simulink model "pendubotG_PID_FUNZY"  (R2017b)
settings: Solver=FixedStepAuto  StartTime=0.0  StopTime=10  FixedStep=0.01  RelTol=1e-3
values from neighbouring files (symbols this model uses):
  Kd1 = par(bestchrom,3)-500    [pidGA.m]    (also in thongso_pid_chuan.m = -214.2; thongso_pid_chuan_phuc_chay.m = -315.3)
  Kp1 = par(bestchrom,1)-500    [pidGA.m]    (also in thongso_pid_chuan.m = -416.5; thongso_pid_chuan_phuc_chay.m = -885.5)
  q1_d_init = 0.0001    [goc_init.m]
  q1_init = pi/2+0.001    (= 1.57179632679)    [goc_init.m]
  q2_d_init = 0.02    [goc_init.m]
  q2_init = 0.007    [goc_init.m]
libraries: fuzblock x4
settings Model: Creator=vohuu  LastModifiedBy=DELL
settings DebuggingCC: UnconnectedInputMsg=none  UnconnectedOutputMsg=none  UnconnectedLineMsg=none  SFMachineParentedDataDiag=error
settings SFSimCC: SimUseLocalCustomCode=on
settings RTWCC: RTWUseLocalCustomCode=on
settings CodeAppCC: StateflowObjectComments=on

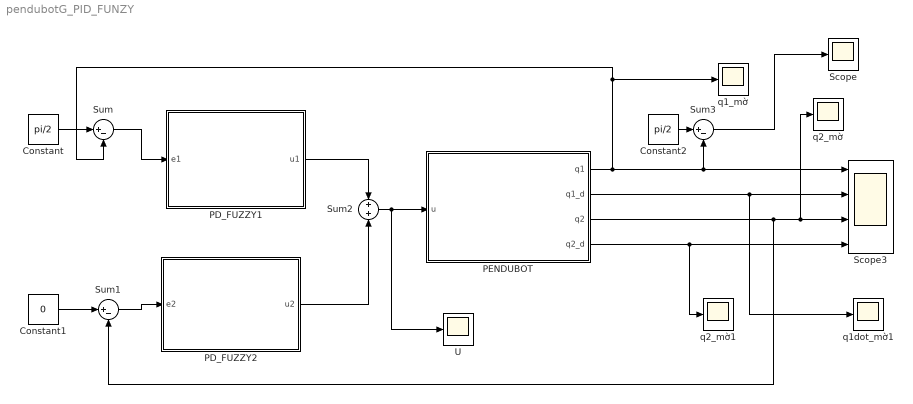
== system pendubotG_PID_FUNZY ==
  Constant : Constant  Value=pi/2
  Constant1 : Constant  Value=0
  Constant2 : Constant  Value=pi/2
  PD_FUZZY1 : Subsystem
  PD_FUZZY2 : Subsystem
  PENDUBOT : Subsystem
  Scope : Scope
  Scope3 : Scope  NumInputPorts=4
  Sum : Sum  Inputs=|+-
  Sum1 : Sum  Inputs=|+-
  Sum2 : Sum
  Sum3 : Sum  Inputs=|+-
  "U " : Scope
  q1_mờ : Scope
  q1dot_mờ1 : Scope
  q2_mờ : Scope
  q2_mờ1 : Scope
  wires:
  Sum1/1 -> PD_FUZZY2/1(e2)
  PD_FUZZY2/1(u2) -> Sum2/2
  Constant1/1 -> Sum1/1
  Sum/1 -> PD_FUZZY1/1(e1)
  PENDUBOT/4(q2_d) -> q2_mờ1/1, Scope3/4
  Sum2/1 -> "U "/1, PENDUBOT/1(u)
  PENDUBOT/2(q1_d) -> q1dot_mờ1/1, Scope3/2
  Constant/1 -> Sum/1
  PENDUBOT/3(q2) -> q2_mờ/1, Scope3/3, Sum1/2
  PENDUBOT/1(q1) -> Scope3/1, Sum3/2, Sum/2, q1_mờ/1
  Constant2/1 -> Sum3/1
  PD_FUZZY1/1(u1) -> Sum2/1
  Sum3/1 -> Scope/1

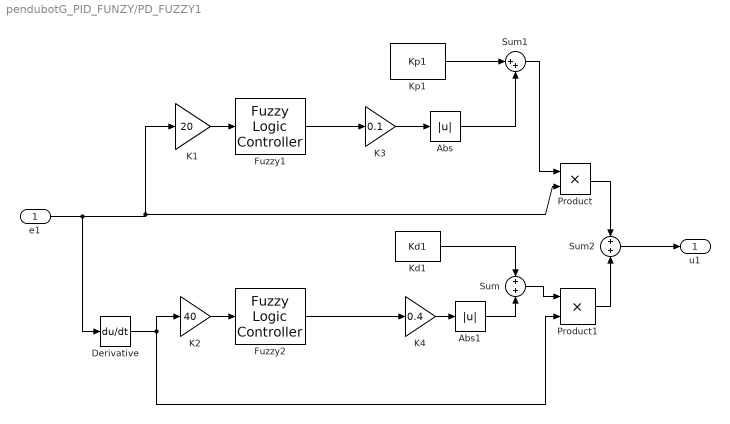
== system pendubotG_PID_FUNZY/PD_FUZZY1 ==
  e1 : Inport
  Abs : Abs
  Abs1 : Abs
  Derivative : Derivative
  "Fuzzy1 " : fuzblock/Fuzzy Logic  Controller  FIS='RULE111.fis'  OutputSampleNumber=101  DataType=double  FuzzifiedInputs=off  RuleFiringStrengths=off  RuleOutputs=off  AggregatedOutputs=off  SimulateUsing=Interpreted execution
  Fuzzy2 : fuzblock/Fuzzy Logic  Controller  FIS='RULE222.fis'  OutputSampleNumber=101  DataType=double  FuzzifiedInputs=off  RuleFiringStrengths=off  RuleOutputs=off  AggregatedOutputs=off  SimulateUsing=Interpreted execution
  K1 : Gain  Gain=20
  K2 : Gain  Gain=40
  K3 : Gain  Gain=0.1
  K4 : Gain  Gain=0.4
  Kd1 : Constant  Value=Kd1
  Kp1 : Constant  Value=Kp1
  Product : Product
  Product1 : Product
  Sum : Sum
  Sum1 : Sum  Inputs=|++
  Sum2 : Sum
  u1 : Outport
  wires:
  K1/1 -> "Fuzzy1 "/1
  "Fuzzy1 "/1 -> K3/1
  K3/1 -> Abs/1
  Kp1/1 -> Sum1/1
  Sum1/1 -> Product/1
  e1/1 -> K1/1, Product/2, Derivative/1
  Abs/1 -> Sum1/2
  K2/1 -> Fuzzy2/1
  Derivative/1 -> Product1/2, K2/1
  Fuzzy2/1 -> K4/1
  Kd1/1 -> Sum/1
  K4/1 -> Abs1/1
  Abs1/1 -> Sum/2
  Sum/1 -> Product1/1
  Product1/1 -> Sum2/2
  Product/1 -> Sum2/1
  Sum2/1 -> u1/1

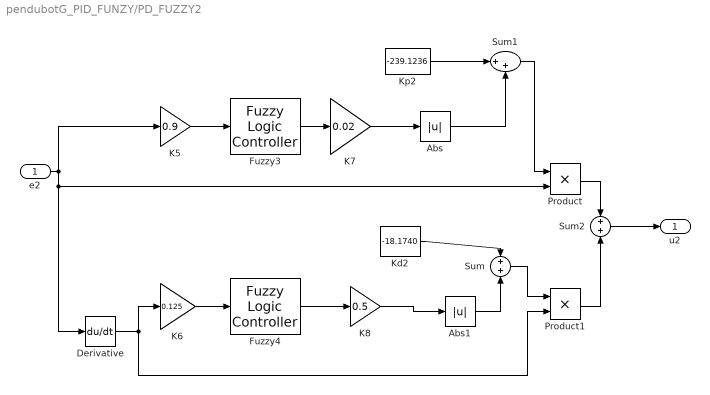
== system pendubotG_PID_FUNZY/PD_FUZZY2 ==
  e2 : Inport
  Abs : Abs
  Abs1 : Abs
  Derivative : Derivative
  Fuzzy3 : fuzblock/Fuzzy Logic  Controller  FIS='RULE333.fis'  OutputSampleNumber=101  DataType=double  FuzzifiedInputs=off  RuleFiringStrengths=off  RuleOutputs=off  AggregatedOutputs=off  SimulateUsing=Interpreted execution
  Fuzzy4 : fuzblock/Fuzzy Logic  Controller  FIS='RULE444.fis'  OutputSampleNumber=101  DataType=double  FuzzifiedInputs=off  RuleFiringStrengths=off  RuleOutputs=off  AggregatedOutputs=off  SimulateUsing=Interpreted execution
  K5 : Gain  Gain=0.9
  K6 : Gain  Gain=0.125
  K7 : Gain  Gain=0.02
  K8 : Gain  Gain=0.5
  Kd2 : Constant  Value=-18.1740
  Kp2 : Constant  Value=-239.1236
  Product : Product
  Product1 : Product
  Sum : Sum
  Sum1 : Sum  Inputs=|++
  Sum2 : Sum
  u2 : Outport
  wires:
  Sum2/1 -> u2/1
  Product/1 -> Sum2/1
  Product1/1 -> Sum2/2
  Sum/1 -> Product1/1
  Abs1/1 -> Sum/2
  K8/1 -> Abs1/1
  Kd2/1 -> Sum/1
  Fuzzy4/1 -> K8/1
  Derivative/1 -> Product1/2, K6/1
  K6/1 -> Fuzzy4/1
  Abs/1 -> Sum1/2
  e2/1 -> Derivative/1, Product/2, K5/1
  Sum1/1 -> Product/1
  Kp2/1 -> Sum1/1
  K7/1 -> Abs/1
  Fuzzy3/1 -> K7/1
  K5/1 -> Fuzzy3/1

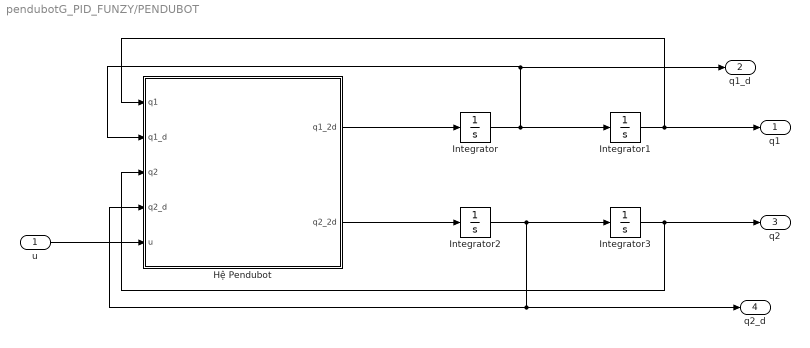
== system pendubotG_PID_FUNZY/PENDUBOT ==
  u : Inport
  Hệ Pendubot : MATLAB Function  TreatAsAtomicUnit=on
  Integrator : Integrator  InitialCondition=q1_d_init
  Integrator1 : Integrator  InitialCondition=q1_init
  Integrator2 : Integrator  InitialCondition=q2_d_init
  Integrator3 : Integrator  InitialCondition=q2_init
  q1 : Outport
  q1_d : Outport  Port=2
  q2 : Outport  Port=3
  q2_d : Outport  Port=4
  wires:
  Integrator2/1 -> q2_d/1, Hệ Pendubot/4(q2_d), Integrator3/1
  Integrator3/1 -> Hệ Pendubot/3(q2), q2/1
  Integrator/1 -> Hệ Pendubot/2(q1_d), q1_d/1, Integrator1/1
  u/1 -> Hệ Pendubot/5(u)
  Hệ Pendubot/2(q2_2d) -> Integrator2/1
  Integrator1/1 -> Hệ Pendubot/1(q1), q1/1
  Hệ Pendubot/1(q1_2d) -> Integrator/1

== matlab function pendubotG_PID_FUNZY/PENDUBOT/Hệ Pendubot ==
  data: q1 input; q1_2d output; q1_d input; q2 input; q2_d input; u input; q2_2d output
function [q1_2d,q2_2d] = fcn(q1,q1_d,q2,q2_d,u)
m1=1.068;
m2=0.07;
l1=0.146;
l2=0.253;
lc1=0.055;
lc2=0.149;
I1=0.0189;
I2=0.000409;
Kb=0.0864;
Kt=0.0864;
Rm=3.7;
Cm=0.000415;
Jm=0.000427;
g=9.80665;
K1=Kt/Rm;
K2=((Kt*Kb)/Rm)+Cm;
K3=Jm;
beta1=m1*lc1^2+m2*l1^2+I1;
beta2=m2*lc2^2+I2;
beta3=m2*l1*lc2;
beta4=m1*lc1+m2*l1;
beta5=m2*lc2;
q1_2d=1/(beta1*beta2-beta3^2*(cos(q2))^2+K3*beta2)*(beta2*beta3*sin(q2)*(q1_d+q2_d)^2+beta3^2*cos(q2)*sin(q2)*q1_d^2-beta2*beta4*g*cos(q1)+beta3*beta5*g*cos(q2)*cos(q1+q2)+beta2*K1*u-K2*beta2*q1_d);
%q2_2d=-(2*beta3^2*q1_d^2*sin(2*q2) + beta3^2*q2_d^2*sin(2*q2) - 2*K2*beta2*q1_d + 2*K1*beta2*u + 2*K3*beta5*g*cos(q1 + q2) + 2*beta1*beta5*g*cos(q1 + q2) - beta3*beta4*g*cos(q1 + q2) + 2*beta3^2*q1_d*q2_d*sin(2*q2) - 2*K2*beta3*q1_d*cos(q2) + 2*K1*beta3*u*cos(q2) - 2*beta2*beta4*g*cos(q1) + beta3*beta5*g*cos(q1) - beta3*beta4*g*cos(q1 - q2) + beta3*beta5*g*cos(q1 + 2*q2) + 2*K3*beta3*q1_d^2*sin(q2) + 2*beta1*beta3*q1_d^2*sin(q2) + 2*beta2*beta3*q1_d^2*sin(q2) + 2*beta2*beta3*q2_d^2*sin(q2) + 4*beta2*beta3*q1_d*q2_d*sin(q2))/(2*K3*beta2 + 2*beta1*beta2 - beta3^2*cos(2*q2) - beta3^2);
q2_2d=-(beta5*g*cos(q1 + q2)*(K3 + beta1 + beta3*cos(q2)) - beta4*g*cos(q1)*(beta2 + beta3*cos(q2)) - K2*q1_d*(beta2 + beta3*cos(q2)) + beta3*sin(q2)*(q1_d + q2_d)^2*(beta2 + beta3*cos(q2)) + K3*beta3*q1_d^2*sin(q2) + beta3*q1_d^2*sin(q2)*(beta1 + beta3*cos(q2)))/(- beta3^2*cos(q2)^2 + K3*beta2 + beta1*beta2) - (K1*u*(beta2 + beta3*cos(q2)))/(- beta3^2*cos(q2)^2 + K3*beta2 + beta1*beta2);
